simulink model "LATC_Test_Calc"  (R2021b)
settings: Solver=FixedStepDiscrete  StartTime=3849.7586  StopTime=3889.7825  FixedStep=0.01  RelTol=1e-3
values from neighbouring files (symbols this model uses):
  P_Global_CharSpd_ms : value not decoded    [PubParsGlobal.sldd]
  P_Global_SteeringAngleRatio : value not decoded    [PubParsGlobal.sldd]
  P_Global_WheelBase_m : value not decoded    [PubParsGlobal.sldd]
  P_LCS_CycleTime = 0.4 0.4 0.4 0.4 0.4 0.4 0.4 0.4 0.4 0.6 0.6 0.6 0.6 0.6 0.6 0.6 0.4 0.4 0.4 0.4 0.4 0.4 0.4 0.4 0.4 0.6 0.6 0.6 0.6 0.6 0.6 0.6 0.4 0.4 0.4 0.4 0.4 0.4 0.4 0.4 0.4 0.6 0.6 0.6 0.6 0.6 0.6 0.6 0.4 0.4 0.4 0.4 0.4 0.4 0.4 0.4 0.4 0.6 0.6 0.6 0.6 0.6 0.6 0.6 0.4 0.4 0.4 0.4 0.4 0.4 0.4 0.4 0.4 0.6 0.6 0.6 0.6 0.6 0.6 0.6 0.4 0.4 0.4 0.4 0.4 0.4 0.4 0.4 0.4 0.6 0.6 0.6 0.6 0.6 0.6 0.6 0.4 0.4 0.4 0.4    [LATC.sldd]
  P_LCS_ESS_AngleSlope_Limit = 2.9    [LATC.sldd]    (also in LCS_v05.sldd)
  P_LCS_LATC_CurOffsetVehicleSpdLimitValue_degs = 7.0    [LATC.sldd]
  P_LCS_LATC_ELKAngleSlope_ratio : value not decoded    [LATC.sldd]
  P_LCS_LATC_ELKMaxLatAcc_ms2 : value not decoded    [LATC.sldd]
  P_LCS_LATC_ESSAngleSlope_ratio : value not decoded    [LATC.sldd]
  P_LCS_LATC_ESSMaxLatAcc_ms2 : value not decoded    [LATC.sldd]
  P_LCS_LATC_LCAngleSlope_ratio : value not decoded    [LATC.sldd]
  P_LCS_LATC_LCCancleMaxLatAcc_ms2 : value not decoded    [LATC.sldd]
  P_LCS_LATC_LCEcoAngleSlope_ratio : value not decoded    [LATC.sldd]
  P_LCS_LATC_LCEcoMaxLatAcc_ms2 : value not decoded    [LATC.sldd]
  P_LCS_LATC_LCKAngleSlope_ratio : value not decoded    [LATC.sldd]
  P_LCS_LATC_LCKIEAngleSlope_ratio : value not decoded    [LATC.sldd]
  P_LCS_LATC_LCKIEMaxLatAcc_ms2 : value not decoded    [LATC.sldd]
  P_LCS_LATC_LCKMaxLatAcc_ms2 : value not decoded    [LATC.sldd]
  P_LCS_LATC_LCNormalAngleSlope_ratio : value not decoded    [LATC.sldd]
  P_LCS_LATC_LCNormalMaxLatAcc_ms2 : value not decoded    [LATC.sldd]
  P_LCS_LATC_LCSportAngleSlope_ratio : value not decoded    [LATC.sldd]
  P_LCS_LATC_LCSportMaxLatAcc_ms2 : value not decoded    [LATC.sldd]
  P_LCS_LATC_LKAAngleSlope_ratio : value not decoded    [LATC.sldd]
  P_LCS_LATC_LKAMaxLatAcc_ms2 : value not decoded    [LATC.sldd]
  P_LCS_LATC_MatrixQ1_st = 0.8 0.8 1.2 1.4 1.4 1.4 2.0 2.2 2.2 2.2 2.2 2.2 2.2 2.2 2.2 2.2 0.8 0.8 1.2 1.4 1.4 1.4 2.0 2.2 2.2 2.2 2.2 2.2 2.2 2.2 2.2 2.2 0.8 0.8 1.2 1.4 1.4 1.4 2.0 2.2 2.2 2.2 2.2 2.2 2.2 2.2 2.2 2.2 0.8 0.8 1.2 1.4 1.4 1.4 2.0 2.2 2.2 2.2 2.2 2.2 2.2 2.2 2.2 2.2 0.8 0.8 1.2 1.4 1.4 1.4 2.0 2.2 2.2 2.2 2.2 2.2 2.2 2.2 2.2 2.2 0.8 0.8 1.2 1.4 1.4 1.4 2.0 2.2 2.2 2.2 2.2 2.2 2.2 2.2 2.2 2.2 0.8 0.8 1.2 1.4    [LATC.sldd]
  P_LCS_LATC_MatrixQ3_st = 20.0 20.0 20.0 20.0 20.0 15.0 15.0 15.0 15.0 15.0 15.0 15.0 15.0 13.0 13.0 13.0 20.0 20.0 20.0 20.0 20.0 15.0 15.0 15.0 15.0 15.0 15.0 15.0 15.0 13.0 13.0 13.0 20.0 20.0 20.0 20.0 20.0 15.0 15.0 15.0 15.0 15.0 15.0 15.0 15.0 13.0 13.0 13.0 20.0 20.0 20.0 20.0 20.0 15.0 15.0 15.0 15.0 15.0 15.0 15.0 15.0 13.0 13.0 13.0 20.0 20.0 20.0 20.0 20.0 15.0 15.0 15.0 15.0 15.0 15.0 15.0 15.0 13.0 13.0 13.0    [LATC.sldd]
  P_LCS_LATC_MatrixR_st = 10.0 10.0 10.0 10.0 10.0 10.0 10.0 15.0 15.0 15.0 15.0 15.0 15.0 15.0 15.0 15.0 10.0 10.0 10.0 10.0 10.0 10.0 10.0 15.0 15.0 15.0 15.0 15.0 15.0 15.0 15.0 15.0 10.0 10.0 10.0 10.0 10.0 10.0 10.0 15.0 15.0 15.0 15.0 15.0 15.0 15.0 15.0 15.0 10.0 10.0 10.0 10.0 10.0 10.0 10.0 15.0 15.0 15.0 15.0 15.0 15.0 15.0 15.0 15.0 10.0 10.0 10.0 10.0 10.0 10.0 10.0 15.0 15.0 15.0 15.0 15.0 15.0 15.0 15.0 15.0    [LATC.sldd]
  P_LCS_LATC_StateActivAngleSlopeLimit_ratio : value not decoded    [LATC.sldd]
  P_LCS_LATC_StateActiveFlg_TabX_st : value not decoded    [LATC.sldd]
  P_LCS_LATC_StateActiveHoldTime_TabY_st : value not decoded    [LATC.sldd]
  P_LCS_LATC_StateHoldTime_st = 250.0    [LATC.sldd]
  P_LCS_LATC_TarAngleFliterWindowSize = 5.0    [LATC.sldd]
  P_LCS_LineVaildSW = 0.0    [LATC.sldd]
  P_LCS_Lookahead_Distance : value not decoded    [LATC.sldd]
  P_LCS_VehicleSpd_TabX_Kph : value not decoded    [LATC.sldd]
libraries: simulink x4
(part 4 of 4)

== matlab function LATC_Test_Calc/LCS_Angle/Controller/StateErrorCalc/Reference_Point_Select/MatchPoint_ProjectPoint ==
  data: CurPosX input; CurPosY input; MatchPtX output; MatchPtY output; MatchPtTheta output; MatchPtCurve output; MatchPtS output; RefTrajX input; ProjectPtX output; ProjectPtY output; RefTrajY input; RefTrajTheta input; RefTrajCurve input; ProjectPtTheta output; ProjectPtCurve output; RefTrajS input; ProjectPtS output
function [MatchPtX,MatchPtY,MatchPtTheta,MatchPtCurve,MatchPtS,ProjectPtX,ProjectPtY,ProjectPtTheta,ProjectPtCurve,ProjectPtS] ...
           = SearchProjectPoint(CurPosX,CurPosY,RefTrajX,RefTrajY,RefTrajTheta,RefTrajCurve,RefTrajS)
PathPtNum = single(length(RefTrajX));
Index = single(1);
MinDis = single(10000);
% 声明increase_count，用于表示在遍历时distance连续增加的个数
increase_count = 0;

for i = 1:PathPtNum
    Dis = sqrt((CurPosX-RefTrajX(i,1))*(CurPosX-RefTrajX(i,1))+(CurPosY-RefTrajY(i,1))*(CurPosY-RefTrajY(i,1)));
    if (Dis < MinDis)
        MinDis = Dis;
        Index = i;
        increase_count = 0;
    else
        increase_count = increase_count + 1;
    end
    %如果distance连续增加20次就不要再遍历了，节省时间
    if increase_count > 20
        break;
    end
end
% 找到匹配点索引MatchPoint
MatchPtX = RefTrajX(Index,1);
MatchPtY = RefTrajY(Index,1);
MatchPtTheta = RefTrajTheta(Index,1);
MatchPtCurve = RefTrajCurve(Index,1);
MatchPtS = RefTrajS(Index,1);
%求解垂直点坐标ProjectPoint
if (Index == 1) %第一个点
    PointEgoX = CurPosX;
    PointEgoY = CurPosY;
    PointA_X = RefTrajX(1,1);
    PointA_Y = RefTrajY(1,1);
    PointB_X = RefTrajX(2,1);
    PointB_Y = RefTrajY(2,1);
    DotProductA = DotProduct(PointA_X,PointA_Y,PointEgoX,PointEgoY,PointB_X,PointB_Y);
    DotProductB = DotProduct(PointB_X,PointB_Y,PointEgoX,PointEgoY,PointA_X,PointA_Y);
    if(DotProductA>=0 && DotProductB>=0)
        IndexA = single(1);
        IndexB = single(2);
    else
        IndexA = single(1);
        IndexB = single(1);
    end
elseif (Index == PathPtNum)%最后一个点
    PointEgoX = CurPosX;
    PointEgoY = CurPosY;
    PointA_X = RefTrajX(PathPtNum-1,1);
    PointA_Y = RefTrajY(PathPtNum-1,1);
    PointB_X = RefTrajX(PathPtNum,1);
    PointB_Y = RefTrajY(PathPtNum,1);
    DotProductA = DotProduct(PointA_X,PointA_Y,PointEgoX,PointEgoY,PointB_X,PointB_Y);
    DotProductB = DotProduct(PointB_X,PointB_Y,PointEgoX,PointEgoY,PointA_X,PointA_Y);
    if(DotProductA>=0 && DotProductB>=0)
        IndexA = PathPtNum-1;
        IndexB = PathPtNum;
    else
        IndexA = PathPtNum;
        IndexB = PathPtNum;
    end
else
    PointEgoX = CurPosX;
    PointEgoY = CurPosY;
    PointA_X = RefTrajX(Index,1);
    PointA_Y = RefTrajY(Index,1);
    PointB_X = RefTrajX(Index+1,1);
    PointB_Y = RefTrajY(Index+1,1);
    DotProductA = DotProduct(PointA_X,PointA_Y,PointEgoX,PointEgoY,PointB_X,PointB_Y);
    DotProductB = DotProduct(PointB_X,PointB_Y,PointEgoX,PointEgoY,PointA_X,PointA_Y);
    if(DotProductA>=0 && DotProductB>=0)
        IndexA = Index;
        IndexB = Index+1;
    else
        IndexA = Index;
        IndexB = Index-1;
    end
end
% 投影点坐标求解
PointA_X = RefTrajX(IndexA,1);
PointA_Y = RefTrajY(IndexA,1);
PointB_X = RefTrajX(IndexB,1);
PointB_Y = RefTrajY(IndexB,1);
[ProjectPtX,ProjectPtY] = Pt2LineProject(PointEgoX,PointEgoY,PointA_X,PointA_Y,PointB_X,PointB_Y);
% 求解投影点的朝向角和曲率
LengthOA = CalTwoPtLength(ProjectPtX,ProjectPtY,PointA_X,PointA_Y);
LengthAB = CalTwoPtLength(PointA_X,PointA_Y,PointB_X,PointB_Y);
if ( LengthAB < 0.001)
    fWeight = single(1);
else
    fWeight = single(LengthOA/LengthAB);
end
ProjectPtTheta = RefTrajTheta(IndexA,1)*fWeight + RefTrajTheta(IndexB,1)*(1-fWeight);
ProjectPtCurve = RefTrajCurve(IndexA,1)*fWeight + RefTrajCurve(IndexB,1)*(1-fWeight);
if IndexA > IndexB
    ProjectPtS =  RefTrajS(IndexA,1) - LengthAB*fWeight;
elseif IndexA < IndexB
    ProjectPtS =  RefTrajS(IndexA,1) + LengthAB*fWeight;
else
    ProjectPtS =  RefTrajS(IndexA,1);
end
end

function DotProduct_Result = DotProduct(X1,Y1,X2,Y2,X3,Y3)
DotProduct_Result = (X2 - X1)*(X3 - X1) + (Y2 - Y1)*(Y3 - Y1);
end
function [ProjectPtX,ProjectPtY] = Pt2LineProject(X,Y,X1,Y1,X2,Y2)
%X = single(0);Y = single(0);X1 = single(0);Y1 = single(0);X2 = single(0);Y2 = single(0);
if (abs((X2-X1)*(X2-X1) + (Y2-Y1)*(Y2-Y1)) > 0.0001)
    ProjectPtX = (X*(X2-X1)*(X2-X1)+Y*(Y2-Y1)*(X2-X1)+(X1*Y2-X2*Y1)*(Y2-Y1))/((X2-X1)*(X2-X1)+(Y2-Y1)*(Y2-Y1));
    ProjectPtY = (X*(X2-X1)*(Y2-Y1)+Y*(Y2-Y1)*(Y2-Y1)+(X2*Y1-X1*Y2)*(X2-X1))/((X2-X1)*(X2-X1)+(Y2-Y1)*(Y2-Y1));
else
    ProjectPtX = X1;
    ProjectPtY = Y1;
end
end
function Length = CalTwoPtLength(X1,Y1,X2,Y2)
Length = sqrt((X1-X2)*(X1-X2) + (Y1-Y2)*(Y1-Y2));
end

== matlab function LATC_Test_Calc/LCS_Angle/Controller/StateErrorCalc/Reference_Point_Select/MATLAB Function1 ==
  data: Pt1X input; Dis output; Pt1Y input; Pt2X input; Pt2Y input; AbsDis output
function [Dis,AbsDis]= fcn(Pt1X,Pt1Y,Pt2X,Pt2Y)
Dis = (sqrt((Pt1X-Pt2X)*(Pt1X-Pt2X)+(Pt1Y-Pt2Y)*(Pt1Y-Pt2Y)))*sign(Pt1Y);
AbsDis = sqrt((Pt1X-Pt2X)*(Pt1X-Pt2X)+(Pt1Y-Pt2Y)*(Pt1Y-Pt2Y));
end

== matlab function LATC_Test_Calc/LCS_Angle/Controller/StateErrorCalc/Reference_Point_Select/MATLAB Function2 ==
  data: path_x output; path_y output; path_x input; path_heading output; path_y input; path_kappa output; path_s output
function [path_x,path_y,path_heading,path_kappa,path_s] = fcn(path_x,path_y)
%该模块是直接采用的老王模型中的通用模块
%该函数将计算path的切线方向与x轴的夹角和曲率
%输入：path_x,y路径坐标
%输出：path heading kappa 路径的heading和曲率
%原理 heading = arctan(dy/dx);
%     kappa = dheading/ds;
%     ds = (dx^2 + dy^2)^0.5

%注意，角度的多值性会带来很大的麻烦，需要慎重处理
%例，x 与 x + 2pi往往代表同一个角度，这种多值性在计算曲率会带来麻烦
%比如 原本是(0.1 - (-0.1))/ds，但如果计算出的-0.1多了一个2pi
%kappa就等于(0.1 - (-0.1 + 2*pi))/ds，曲率会变得非常大
%还有若采用中点欧拉法计算heading时，(即使用(y2 - y1)/(x2 - x1)的反正切计算一个角度 ，用(y1 - y0)/(x1
%-x0)的反正切又计算一个角度，然后加起来除以2),如果精确值是 (a1 + a2)/2,但最终计算的结果可能是(a1 + a2 + 2pi)/2
% 还有 tan(x) = tan(x + pi) 所以arctan(tan(x))可能等于x，也可能等于x + pi
% 角度的处理非常麻烦，而且角度处理不当往往是许多奇怪错误的源头

dx = diff(path_x);
dy = diff(path_y);
%用中点欧拉法要比向前欧拉法向后欧拉法更精确，但是也可能计算出的结果比精确值多一个pi
%在这里对dx,dy做中点欧拉法，使用四象限反正切计算角度
dx_pre = [dx(1);dx];
dx_after = [dx;dx(end)];
dx_final = (dx_pre + dx_after)/2;

dy_pre = [dy(1);dy];
dy_after = [dy;dy(end)];
dy_final = (dy_pre + dy_after)/2;

ds_final = sqrt(dx_final.^2 + dy_final.^2);
cum_ds = cumsum(ds_final);
path_heading = atan2(dy_final,dx_final);

dheading = diff(path_heading);
dheading_pre = [dheading(1);dheading];
dheading_after = [dheading;dheading(end)];
dheading_final = (dheading_pre + dheading_after) / 2;
%为了防止dheading出现多一个2pi的错误，假设真实的dheading较小，用sin(dheading)近似dheading
path_kappa = sin(dheading_final) ./ ds_final;
path_s = single(zeros(length(path_x),1));
path_s(2:end,1) = cum_ds(1:end-1,1);
end

== matlab function LATC_Test_Calc/LCS_Angle/Controller/StateErrorCalc/EgoMovement ==
  data: dDeltaX output single size=1; dDeltaY output single size=1; tCycle input single size=1; CosOfPsi output single size=1; Kap input single size=1; psiDtOptSync input single size=1; Vego input single size=1; alpSideSlipAngle input single size=1; SinOfPsi output single size=1; ego_x input; ego_y input; ego_heading input; predict_x output; predict_y output; predict_heading output; predict_spd output; predict_yawrate output
function [dDeltaX,dDeltaY,CosOfPsi,SinOfPsi,predict_x,predict_y,predict_heading,predict_spd,predict_yawrate] = EgoVehicleMovement(tCycle,Kap,psiDtOptSync,Vego,alpSideSlipAngle,ego_x,ego_y,ego_heading)
%#codegen
if Kap==0
    dDeltaX = Vego*tCycle;
    dDeltaY = single(0);
    CosOfPsi = single(1);
    SinOfPsi = single(0);
else
    t_kap = Kap;
    if ((Kap>0.125)||(Kap<-0.125))&&(Vego>1)
        t_kapPsiDtSync = psiDtOptSync/Vego;      %实际计算的曲率
        if abs(t_kapPsiDtSync)>abs(Kap)          
            t_kap = t_kapPsiDtSync;
        end
    end
    t_Psi = t_kap*Vego*tCycle;
    SinOfPsi = sin(t_Psi);
    CosOfPsi = cos(t_Psi);
    t_dDeltaXTemp = SinOfPsi/t_kap;
    t_dDeltaYTemp = 2*(sin(t_Psi/2)*sin(t_Psi/2))/t_kap;
    dDeltaX = cos(alpSideSlipAngle)*t_dDeltaXTemp - sin(alpSideSlipAngle)*t_dDeltaYTemp;
    dDeltaY = sin(alpSideSlipAngle)*t_dDeltaXTemp + cos(alpSideSlipAngle)*t_dDeltaYTemp;
end
predict_x = ego_x + dDeltaY; % 车辆运动推算坐标系是在车辆坐标系下进行，规划与控制坐标系是在常规直角坐标系
predict_y = ego_y + dDeltaX;
predict_heading = ego_heading; % 暂时认为朝向角不变，调试或者仿真时得看看把实际变化的角度考虑进来
predict_spd = Vego;
predict_yawrate = psiDtOptSync;
end

== matlab function LATC_Test_Calc/LCS_Angle/Controller/Understeer&Offset_Calc/YOD_Ackman ==
  data: AckConst output; VxvRef input; Vch input; WheelBase input; AlpWheelAngle input; PsiDtAckK1 input single; PsiDtAck output
function [AckConst,PsiDtAck] = Ackman(VxvRef,Vch,WheelBase,AlpWheelAngle,PsiDtAckK1)
%#codegen
if VxvRef==uint8(0)%转换常数数据类型
    PsiDtAckRaw = single(0);%转换常数数据类型
    AckConst = single(1);%转换常数数据类型
else
    AckConst = min((single(1)+VxvRef*VxvRef/(Vch*Vch))*WheelBase/VxvRef,single(32767));%转换常数数据类型
    PsiDtAckRaw = AlpWheelAngle/AckConst;
end
PsiDtAck = (single(0.02/0.1))*(PsiDtAckRaw-PsiDtAckK1)+PsiDtAckK1;%转换常数数据类型

== matlab function LATC_Test_Calc/LCS_Angle/Controller/TargetAngleCalc/TarSteerAngleCalc ==
  data: steer_angle_cmd_temp output; steer_feedforward_temp output; steer_feedbackward_temp output; steer_limit_temp output; LatError_contribution output; LatErrorRate_contribution output; HeadingError_contribution output; HeadingErrorRate_contribution output; ControlValid input; SteerAngle input; steer_angle output size=[1,1]; Veh_Speed input; ref_curvature input; lateral_error input; lateral_error_rate input; heading_error input; heading_error_rate input; Left_steer_ratio input; Right_steer_ratio input; Matrix_q1 input; Matrix_q3 input; Matrix_R input; Max_lateral_acceleration input; TarSteerAngleSlope input; CurrentSteerAngleOffset input; steer_angleK1 input single
function [steer_angle_cmd_temp,steer_feedforward_temp,steer_feedbackward_temp,steer_limit_temp,...
    LatError_contribution,LatErrorRate_contribution,HeadingError_contribution,HeadingErrorRate_contribution,steer_angle]= LQR_Algorithm(ControlValid,SteerAngle,Veh_Speed,ref_curvature,lateral_error,lateral_error_rate,heading_error,heading_error_rate,...
    Left_steer_ratio,Right_steer_ratio,Matrix_q1,Matrix_q3,Matrix_R,Max_lateral_acceleration,TarSteerAngleSlope,CurrentSteerAngleOffset,steer_angleK1)
if ControlValid
    %% 1.车辆参数
    %1.1 车的大小及长度参数
    veh_params.vehicle_length = single(4.875);
    veh_params.vehicle_width  = single(2.2);
    veh_params.vehicle_height = single(1.69);
    %1.2 车辆控制参数
    veh_params.wheel_base = single(2.92);               %轴距, m
    veh_params.Vch = single(23.5);                      %特征车速
    veh_params.max_steer_angle = single(53 / 180 * pi); %前轮最大转角
    veh_params.max_acceleration = single(2);            %车辆最大加速度
    veh_params.max_deceleration = single(-2);           %车辆最大减速度
    veh_params.left_steer_ratio = Left_steer_ratio;     %车辆左侧转向传动比%
    veh_params.right_steer_ratio = Right_steer_ratio;   %车辆右侧转向传动比%
    veh_params.cf = single(155494.663);                 %车辆前轮侧偏刚度
    veh_params.cr = single(155494.663);                 %车辆后轮侧偏刚度 
    veh_params.mass_fl = single(520);                   %车辆左前轮负重
    veh_params.mass_fr = single(520);                   %车辆右前轮负重
    veh_params.mass_rl = single(520);                   %车辆左后轮负重
    veh_params.mass_rr = single(520);                   %车辆右后轮负重
    %% 2.控制参数计算
    mass_front =  veh_params.mass_fl + veh_params.mass_fr;
    mass_rear  =  veh_params.mass_rl + veh_params.mass_rr;
    mass =  mass_front + mass_rear;
    lf = veh_params.wheel_base * (single(1.0) - mass_front / mass);
    lr = veh_params.wheel_base * (single(1.0) - mass_rear / mass);
    iz = lf * lf * mass_front + lr * lr * mass_rear;
    %% 3.LQR参数设置
    lqr_eps = single(0.01);    %最小精度
    lqr_max_iteration = single(800);    %最大迭代次数
    
    basic_state_size = uint8(4);
    control_size = uint8(1);
    
    matrix_a=  single(zeros(basic_state_size,basic_state_size));
    matrix_a_coeff = single(zeros(basic_state_size,basic_state_size));
    I = single(eye(basic_state_size,basic_state_size));
    matrix_a(1,2) = single(1.0);
    matrix_a(2,3) = single((veh_params.cf + veh_params.cr ) / mass);
    matrix_a(3,4) = single(1.0);
    matrix_a(4,3) = single((lf * veh_params.cf - lr * veh_params.cr) / iz);
    
    matrix_a_coeff(2,2) = single(-(veh_params.cf + veh_params.cr) / mass);
    matrix_a_coeff(2,4) = single((lr * veh_params.cr - lf * veh_params.cf) / mass);
    matrix_a_coeff(3,4) = single(1.0);
    matrix_a_coeff(4,2) = single((lr * veh_params.cr - lf * veh_params.cf) / iz);
    matrix_a_coeff(4,4) = single(-1.0 * (lf * lf * veh_params.cf + lr * lr * veh_params.cr)/iz);
    
    matrix_a(2,2) = matrix_a_coeff(2,2);
    matrix_a(2,4) = matrix_a_coeff(2,4);
    matrix_a(4,2) = matrix_a_coeff(4,2);
    matrix_a(4,4) = matrix_a_coeff(4,4);
    
    matrix_b = single(zeros(basic_state_size,control_size));
    matrix_b(2,1) = veh_params.cf/mass;
    matrix_b(4,1) = lf * veh_params.cf /iz;
    
    matrix_q = single(zeros(4,4));
    matrix_q(1,1) = Matrix_q1;                      %调整q矩阵的第一、三个参数，改善转向性能0.0001,0.02  Q为状态权重系数
    matrix_q(3,3) = Matrix_q3;
    matrix_r = single(zeros(1,1));
    matrix_r = Matrix_R;                            %R为控制量权重系数
    
    lqr_params.A = matrix_a;
    lqr_params.B = matrix_b;
    lqr_params.I = I;
    lqr_params.ts = single(0.02);
    lqr_params.lr = lr;
    lqr_params.lf = lf;
    lqr_params.cf=veh_params.cf;
    lqr_params.cr=veh_params.cf;
    lqr_params.iz=iz;
    lqr_params.mass=mass;
    lqr_params.Q =matrix_q ;
    lqr_params.R = matrix_r;
    lqr_params.eps=lqr_eps;
    lqr_params.max_iteration=lqr_max_iteration;
    %% 4.计算前轮转角
    lqr_params.A(2,2) = lqr_params.A(2,2)/(max(Veh_Speed, single(0.2)));
    lqr_params.A(2,4) = lqr_params.A(2,4)/(max(Veh_Speed, single(0.2)));
    lqr_params.A(4,2) = lqr_params.A(4,2)/(max(Veh_Speed, single(0.2)));
    lqr_params.A(4,4) = lqr_params.A(4,4)/(max(Veh_Speed, single(0.2)));
    
    A=lqr_params.A;
    B=lqr_params.B;
    I=lqr_params.I;
    ts=lqr_params.ts;      %控制周期
    min_tol = lqr_params.eps;    %0.01
    max_iter = lqr_params.max_iteration;   %800
    matrix_Q = lqr_params.Q;
    matrix_R = lqr_params.R;
    
    matrix_ad=single(zeros(size(A)));   %4*4零矩阵
    matrix_ad=(I+ts*single(0.5) * A) / (I-ts*single(0.5) * A);  %离散化 
    
    matrix_bd=single(zeros(size(B)));
    matrix_bd=B*ts;
    matrix_k = SolveLQRProblem(matrix_ad, matrix_bd, matrix_Q,matrix_R, min_tol, max_iter);  %求解最优解K
    %% 横向状态变量
    
    matrix_state = single(zeros(4, 1));
    matrix_state(1, 1) = lateral_error;                   %横向误差
    matrix_state(2, 1) = lateral_error_rate;              %横向误差率
    matrix_state(3, 1) = heading_error;                   %航向误差
    matrix_state(4, 1) = heading_error_rate;              %航向误差率
    steer_feedbackward = -(matrix_k * matrix_state);      %反馈控制器
    % 前馈转角
    kv = lqr_params.lr * lqr_params.mass / single(1) / lqr_params.cf / veh_params.wheel_base - ...
        lqr_params.lf * lqr_params.mass / single(1) / lqr_params.cr / veh_params.wheel_base;
    steer_feedforward = (veh_params.wheel_base * ref_curvature + kv * Veh_Speed * Veh_Speed * ref_curvature - matrix_k(1, 3) * ...
        (lqr_params.lr * ref_curvature - lqr_params.lf * lqr_params.mass * Veh_Speed * Veh_Speed * ref_curvature / single(1) / lqr_params.cr / veh_params.wheel_base));%弧度制角度rad
    % 4.3 计算期望前轮偏角
    steer_cmd = steer_feedforward + steer_feedbackward;
    
    if (steer_cmd>=0)
        steer_transmission_ratio = veh_params.left_steer_ratio;
    else
        steer_transmission_ratio = veh_params.right_steer_ratio;
    end 
    LatError_contribution = -matrix_k(1,1) *matrix_state(1, 1) * single(57.3) * steer_transmission_ratio;%横向偏差贡献量，通过观察这几个值调试q1 q3
    LatErrorRate_contribution = -matrix_k(1,2) *matrix_state(2, 1) * single(57.3) * steer_transmission_ratio;%横向偏差贡献量，通过观察这几个值调试q1 q3
    HeadingError_contribution = -matrix_k(1,3) *matrix_state(3, 1) * single(57.3) * steer_transmission_ratio;%横向偏差贡献量，通过观察这几个值调试q1 q3
    HeadingErrorRate_contribution = -matrix_k(1,4) *matrix_state(4, 1) * single(57.3) * steer_transmission_ratio;%横向偏差贡献量，通过观察这几个值调试q1 q3
    
    steer_feedforward_temp = steer_feedforward * single(57.3) * steer_transmission_ratio;%反算方向盘转角并转换为角度制deg
    steer_feedbackward_temp = steer_feedbackward * single(57.3) * steer_transmission_ratio;%反算方向盘转角并转换为角度制deg
    steer_angle_cmd = steer_cmd * single(57.3) * steer_transmission_ratio;%反算方向盘转角并转换为角度制deg
    steer_angle_cmd_temp = steer_angle_cmd;%输出算法计算角度作为观测，最终请求角度会补偿转向不足。
    %% 5.限制期望前轮偏角
    % 5.1 根据横向加速度限制前轮转角
    if Veh_Speed < 1
        steer_limit = atan( Max_lateral_acceleration * veh_params.wheel_base /(Veh_Speed *Veh_Speed))* single(57.3) * steer_transmission_ratio; % 高速计算不准确，更改为下面特征车速计算方法
    else
        AckConst = min((single(1)+Veh_Speed*Veh_Speed/(veh_params.Vch*veh_params.Vch))*veh_params.wheel_base/max(single(1),Veh_Speed),single(32767));
        % PsiDtAckRaw = (SteerAngle/steer_transmission_ratio)/AckConst;
        steer_limit = ((Max_lateral_acceleration * AckConst)/Veh_Speed)* single(57.3) * steer_transmission_ratio;
    end
    %     steer_limit = atan( Max_lateral_acceleration * veh_params.wheel_base /(Veh_Speed *Veh_Speed)) * steer_transmission_ratio;
    steer_angle_cmd = min(steer_limit, max(-steer_limit,steer_angle_cmd));%方向盘角度制deg
    
    steer_angle_deg = steer_angle_cmd + CurrentSteerAngleOffset;
    steer_limit_temp = steer_limit;
    % 5.2 限制方向盘转速
    steer_angle = min(steer_angleK1 + TarSteerAngleSlope,max(steer_angleK1 - TarSteerAngleSlope,steer_angle_deg));
    
else
    steer_angle = SteerAngle;
    steer_angle_cmd_temp = single(0);
    steer_feedforward_temp = single(0);
    steer_feedbackward_temp = single(0);
    steer_limit_temp = single(0);
    LatError_contribution = single(0);
    LatErrorRate_contribution = single(0);
    HeadingError_contribution = single(0);
    HeadingErrorRate_contribution = single(0);
end
end
function ptr_K = SolveLQRProblem(A,B,Q,R,tolerance,max_num_iteration)
  if (size(A,1) ~= size(A,2) || size(B,1) ~= size(A,1) || size(Q,1) ~= size(Q,2) ||size(Q,1) ~= size(A,1) ||size(R,1) ~=size(R,2) || size(R,1) ~=  size(B,2)) 
    ptr_K = single(zeros(1, 4));
    return;
  end
  AT = transpose(A);
  BT = transpose(B);
  P = Q;
  num_iteration = uint8(0);
  % diff = realmax('double');
  diff = realmax('single');
  while (num_iteration < max_num_iteration && diff > tolerance)
    P_next = AT * P * A - AT * P * B / (R + BT * P * B) * BT * P * A + Q;
    diff = abs(max(max(P_next - P)));
    P = P_next;
    num_iteration = num_iteration + uint8(1);
  end
  if (num_iteration >= max_num_iteration)
      ptr_K= single(zeros(1, 4));
  else
      ptr_K = (R + BT * P * B) \ BT * P * A;
  end
end

== matlab function LATC_Test_Calc/LCS_Angle/Trajectory_Planning/QP_Path/generate convex space ==
  data: dp_path_s input; l_min output; dp_path_l input; static_obs_s_set input; static_obs_l_set input; static_obs_length input; static_obs_width input; l_max output
function [l_min,l_max] = fcn(dp_path_s,dp_path_l,static_obs_s_set,static_obs_l_set,static_obs_length,static_obs_width)
    % 该函数将输出每个离散的dp_path_s所对应的l的边界lmin lmax (本质上是质点的凸空间)
    % 输入 动态规划曲线 dp_path_s,dp_path_l
    %      障碍物中心的s l 坐标 static_obs_s,static_obs_l
    %      障碍物的长宽 static_obs_length,static_obs_width 
    % 输出 l_min lmax l 的上下界

    % 输出初始化
    l_min = ones(60,1) * -8;
    l_max = ones(60,1) * 8;
    % 对每个障碍物做遍历
    for i = 1:length(static_obs_s_set)
        if isnan(static_obs_s_set(i))
            break;
        end
        % 计算障碍物的头部和尾部的s
        obs_s_min = static_obs_s_set(i) - static_obs_length/2;
        obs_s_max = static_obs_s_set(i) + static_obs_length/2;
        % 找到dp_path_s 中，与s_head s_end最近的s的编号
        start_index = FindNearIndex(dp_path_s,obs_s_min);
        end_index = FindNearIndex(dp_path_s,obs_s_max);
        path_l = (dp_path_l(start_index) + dp_path_l(end_index))/2;
        if start_index == 1 && end_index == 1
            continue;
        end
        if path_l > static_obs_l_set(i)
            % 意味着决策为向左绕过障碍物
            for j = start_index:end_index
                % l_min(j) 为所有决策为向左绕过障碍物的l边界的最大值
                l_min(j) = max(l_min(j) , static_obs_l_set(i) + static_obs_width/2);
            end
        else
            % 意味着决策为向右绕过障碍物
            for j = start_index:end_index
                % l_max(j) 为所有决策为向右绕过障碍物的l边界的最小值
                l_max(j) = min(l_max(j) , static_obs_l_set(i) - static_obs_width/2);
            end
        end       
    end
end

function y = FindNearIndex(dp_path_s,obs_s)
    % 该函数将找到dp_path_s的所有点中，距离obs_s最近的点的编号
    % 这里要注意obs_s 是在完整的reference line上投影所得到的坐标，所以obs_s可能是负值，也可能会超过dp_path_s最远的长度
    if dp_path_s(1) >= obs_s
        %障碍物在后面
        y = 1;
        return;
    elseif dp_path_s(end) <= obs_s
        y = 60;
        return;
    else
        index = 1;
        while dp_path_s(index) < obs_s
            index = index + 1;
        end
        % 循环退出的条件是dp_path_s(index) >= obs_s 判断一下index 和 index-1哪个离的近
        if dp_path_s(index) - obs_s > obs_s - dp_path_s(index - 1)
            y = index - 1;
        else
            y = index;
        end
    end
end

== matlab function LATC_Test_Calc/LCS_Angle/Controller/TargetAngleCalc/SteerAngSlopeCalc/MATLAB Function3 ==
  data: delytime input uint16; TarDangerLevel input uint8; TarDangerLevelK1 input uint8; FLg output uint8; FLgK1 input uint8; CntK1 input uint16; Cnt output uint16
function [FLg,Cnt] = AngSlopeCalc(delytime,TarDangerLevel,TarDangerLevelK1,FLgK1,CntK1)

Cnt = min(CntK1 + uint16(1),delytime);
if Cnt== delytime
    FLg = uint8(0);
else
    FLg = FLgK1;
end
%FLg = FLgK1;
%% 
if TarDangerLevel==uint8(1) && TarDangerLevelK1==0  % NO function 2 LCK (TarDangerLevelK1==0)
    Cnt =uint16(0);
    FLg = uint8(1);
end

if  TarDangerLevel==uint8(3) && (TarDangerLevelK1==uint8(1)||TarDangerLevelK1==uint8(2)) % LCK/IE 2 LC_Normal
    Cnt =uint16(0);
    FLg = uint8(2);
end

if  TarDangerLevel==uint8(7) && (TarDangerLevelK1==uint8(1)||TarDangerLevelK1==uint8(2)) % LCK/IE 2 LC_Eco
    Cnt =uint16(0);
    FLg = uint8(3);
end

if  TarDangerLevel==uint8(8) && (TarDangerLevelK1==uint8(1)||TarDangerLevelK1==uint8(2)) % LCK/IE 2 LC_sport
    Cnt =uint16(0);
    FLg = uint8(4);
end
if  TarDangerLevel==uint8(6) && (TarDangerLevelK1==uint8(1)||TarDangerLevelK1==uint8(2)) % LCK/IE 2 ESS 后期添加配和ESS Slope 一起调试
    Cnt =uint16(0);
    FLg = uint8(5);
end

== matlab function LATC_Test_Calc/LCS_Angle/Trajectory_Planning/MATLAB Function1 ==
  data: X input; y output; Y input
function y = fcn(X,Y)

y = zeros(length(X),9);
for i = 1:1:length(X)
    y(i,1) = X(i);
    y(i,2) = Y(i);
    y(i,3) = 0;
    y(i,4) = 0;
    y(i,5) = 1;
    y(i,6) = i;
    y(i,7) = 0;
    y(i,8) = 1;
end
end

== matlab function LATC_Test_Calc/LCS_Angle/Trajectory_Planning/DP_Path/increase DP path nodes ==
  data: dp_path_s_init input; dp_path_s_final output; dp_path_l_init input; plan_start_s input; plan_start_l input; plan_start_dl input; plan_start_ddl input; dp_path_l_final output; dp_path_dl_final output; dp_path_ddl_final output
function [dp_path_s_final,dp_path_l_final,dp_path_dl_final,dp_path_ddl_final] = ...
    fcn(dp_path_s_init,dp_path_l_init,plan_start_s,plan_start_l,plan_start_dl,plan_start_ddl)
% 该函数将增密dp_path_s,dp_path_l
% 由于事先不知道动态规划采样的行和列，也就不知道动态规划计算的曲线有多长，因此需要做缓冲
% 每1“米”采样一个点，一共采60个
ds = single(1);
% 输出初始化
Pt_Num = single(60);
dp_path_s_final = single(ones(Pt_Num,1)*nan);
dp_path_l_final = single(ones(Pt_Num,1)*nan);
dp_path_dl_final = single(ones(Pt_Num,1)*nan);
dp_path_ddl_final = single(ones(Pt_Num,1)*nan);

% 设置五次多项式的起点
start_s = plan_start_s;
start_l = plan_start_l;
start_dl = plan_start_dl;
start_ddl = plan_start_ddl;

% 由于不知道有多少个点需要采集，又不能使用动态数组，先定义一个大矩阵300*0.5
l_temp = single(zeros(1,300));
dl_temp = single(zeros(1,300));
ddl_temp = single(zeros(1,300));
% 由于不知道每次取多少点，定义一个局部变量存上一次的点数
persistent Pt_Num_CountK1;
Pt_Num_CountK1=single(0);

for i = 2:length(dp_path_s_init)
    if dp_path_s_init(i) == -1
        break;
    end
    for j=1:10000
        %采样s
        s_node = start_s + ds*(j - 1);
        if s_node >= dp_path_s_init(i)
            break;
        end
    end
    s_cur = single(linspace(start_s,s_node,j));
    end_s = dp_path_s_init(i);
    end_l = dp_path_l_init(i);
    end_dl = single(0);
    end_ddl = single(0);
    coeff = CalcQuinticCoeffient(start_l,start_dl,start_ddl,end_l,end_dl,end_ddl,start_s,end_s);
    a0 = coeff(1);
    a1 = coeff(2);
    a2 = coeff(3);
    a3 = coeff(4);
    a4 = coeff(5);
    a5 = coeff(6);
    l = a0 * ones(1,length(s_cur)) + a1 * s_cur + a2 * s_cur.^2 + a3 * s_cur.^3 +...
        a4 * s_cur.^4 + a5 * s_cur.^5;
    dl = a1 * ones(1,length(s_cur)) + 2 * a2 * s_cur + 3 * a3 * s_cur.^2 + ...
        4 * a4 * s_cur.^3 + 5 * a5 * s_cur.^4;
    ddl = 2 * a2 * ones(1,length(s_cur)) + 6 * a3 * s_cur + 12 * a4 * s_cur.^2 + ...
        20 * a5 * s_cur.^3;

    % 将计算结果存起来
    for ii=1:length(s_cur)
        l_temp(1,ii+Pt_Num_CountK1) = l(1,ii);
        dl_temp(1,ii+Pt_Num_CountK1) = dl(1,ii);
        ddl_temp(1,ii+Pt_Num_CountK1) = ddl(1,ii);
    end
    
    Pt_Num_CountK1 = Pt_Num_CountK1 + single(length(s_cur));
    % end的值赋值给start 做下一步循环
    start_s = end_s;
    start_l = end_l;
    start_dl = end_dl;
    start_ddl = end_ddl;
end

for k = 1:length(l_temp)
    if k == 61
        break;
    end
    dp_path_s_final(k) = plan_start_s + ds * (k - 1);
    dp_path_l_final(k) = l_temp(k);
    dp_path_dl_final(k) = dl_temp(k);
    dp_path_ddl_final(k) = ddl_temp(k);
end
end

function coeff = CalcQuinticCoeffient(start_l,start_dl,start_ddl,end_l,end_dl,end_ddl,start_s,end_s)
    % l = a0 + a1*s + a2*s^2 + a3*s^3 + a4*s^4 + a5*s^5
    % l' = a1 + 2 * a2 * s + 3 * a3 * s^2 + 4 * a4 * s^3 + 5 * a5 * s^4
    % l'' = 2 * a2 + 6 * a3 * s + 12 * a4 * s^2 + 20 * a5 * s^3
    start_s2 = start_s * start_s;
    start_s3 = start_s2 * start_s;
    start_s4 = start_s3 * start_s;
    start_s5 = start_s4 * start_s;
    end_s2 = end_s * end_s;
    end_s3 = end_s2 * end_s;
    end_s4 = end_s3 * end_s;
    end_s5 = end_s4 * end_s;
    A = [1,start_s, start_s2,     start_s3,     start_s4,      start_s5;
         0 1,       2 * start_s,  3 * start_s2, 4 * start_s3,  5 * start_s4;
         0 0,       2,            6 * start_s,  12 * start_s2, 20 * start_s3;
         1,end_s, end_s2,     end_s3,     end_s4,      end_s5;
         0,1,     2 * end_s,  3 * end_s2, 4 * end_s3,  5 * end_s4;
         0,0,     2,          6 * end_s,  12 * end_s2, 20 * end_s3;];
    B = [start_l;
         start_dl;
         start_ddl;
         end_l;
         end_dl;
         end_ddl;];
     coeff = A \ B;
end

== matlab function LATC_Test_Calc/LCS_Angle/Trajectory_Planning/MATLAB Function ==
  data: Ref_X input; TarTraj_x output; Ref_Y input; Plan_Traj_S input; Plan_Traj_L input; VehSpd input; TarTraj_y output; TarTraj_theta output; TarTraj_kappa output
function [TarTraj_x, TarTraj_y, TarTraj_theta, TarTraj_kappa]= ReferenceTrajectory(Ref_X,Ref_Y,Plan_Traj_S,Plan_Traj_L,VehSpd)
rx = single(-1.*Ref_Y);
ry = Ref_X;
waypoints = [rx,ry];
referencePathPointNum = 100; %参考轨迹的点的个数(参考点的分辨率)，此参数会影响最终目标轨迹线的形状，太小会出现轨迹线拐点
referencePath = FrenentReferencePath(waypoints,referencePathPointNum);
%% 将Frenet坐标系下规划的路径转换到直角坐标系中
GtNumTarpoints = 80;
FrenetState = [Plan_Traj_S,Plan_Traj_L];
globalStates = referencePath.frenet2global1D(FrenetState,GtNumTarpoints);
TarTraj_x = single(zeros(GtNumTarpoints,1));TarTraj_y = single(zeros(GtNumTarpoints,1));
TarTraj_theta = single(zeros(GtNumTarpoints,1));TarTraj_kappa = single(zeros(GtNumTarpoints,1));
TarTraj_x = globalStates(:,1);
TarTraj_y = globalStates(:,2);
TarTraj_theta = globalStates(:,3);
TarTraj_kappa = globalStates(:,4);
end
